simulink model "pplace_d"  (Simulink 5.0)
settings: Solver=ode45  StartTime=0.0  StopTime=50.0  RelTol=1e-3
values from neighbouring files (symbols this model uses):
  A = [1 1 1]    [endsem_06.m]    (also in ibm_pp_sat.m = [1 -0.43]; windup.m = [1 -0.7])
  B = [1 2]    [endsem_06.m]    (also in ibm_pp_sat.m = 0.47; windup.m = [1 -0.8])
  R = 1    [ball_im.m]    (also in ball_opt.m; ball_psi.m; pp_im_high.m = conv(Bg,R1); pp_opt.m = conv(Bg,R1))
  S = conv(Ag,S1)    [pp_im_high.m]    (also in pp_opt.m; pp_psi-sav.m)
  st = 0.0001    [ball_im.m]    (also in ball_opt.m; ball_psi.m; comb.m = 1; endsem_06.m = 1)
  t0 = 0    [comb.m]
  Ts = 0.01; [B,A,k] = myc2d(G,Ts)    [ball_im.m]    (also in ball_opt.m; ball_psi.m; comb.m = 0.001; endsem_06.m = 1)
undefined symbols (not defined in the file or in its folder): zk
settings Model: Creator=kannanm  LastModifiedBy=kannan  ExtModeAutoUpdateStatusClock=off

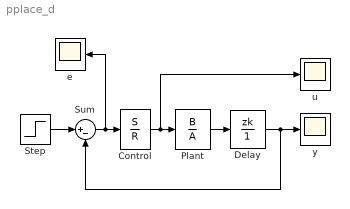
== system pplace_d ==
  Control : DiscreteFilter  Numerator=S  Denominator=R  SampleTime=Ts
  Delay : DiscreteFilter  Numerator=zk  Denominator=1  SampleTime=Ts
  Plant : DiscreteFilter  Numerator=B  Denominator=A  SampleTime=Ts
  Step : Step  Time=t0  After=st  SampleTime=Ts
  Sum : Sum  Inputs=|+-  SaturateOnIntegerOverflow=on
  e : Scope
      settings: SaveName=ScopeData2
  u : Scope
  y : Scope
  wires:
  Step/1 -> Sum/1
  Sum/1 -> Control/1, e/1
  Delay/1 -> y/1, Sum/2
  Plant/1 -> Delay/1
  Control/1 -> Plant/1, u/1
